simulink model "pendulum"  (R2022b)
settings: Solver=VariableStepAuto  StartTime=0.0  StopTime=100  RelTol=1e-3
StartFcn:
  | OpenAnimation;
undefined symbols (not defined in the file or in its folder): figId
libraries: aerolibanimutils x1
settings Model: Creator=l.ribeiro-lustosa  LastModifiedBy=fades
settings DebuggingCC: UnconnectedInputMsg=warning  UnconnectedOutputMsg=warning  UnconnectedLineMsg=warning
settings ModelReferenceCC: EnableRefExpFcnMdlSchedulingChecks=on
settings RTWCC: DLArmComputeVersion=19.05

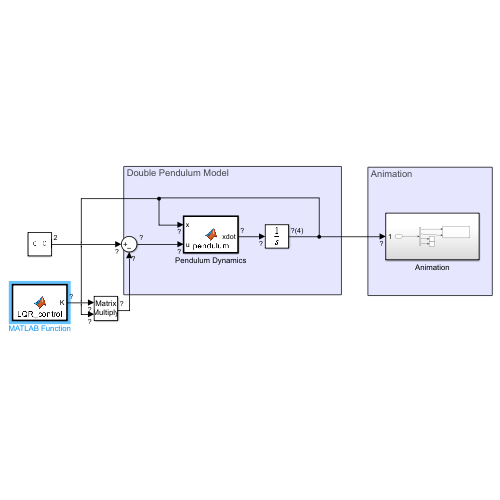
[thumbnail: Simulink's stored preview of the top-level diagram]
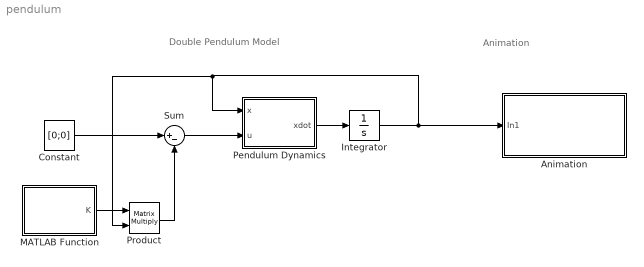
== system pendulum ==
  note: Animation
  note: Double Pendulum Model
  Animation : Subsystem
  Constant : Constant  Value=[0;0]
  Integrator : Integrator  InitialCondition=[175*pi/180;-5*pi/180;0;0]
  MATLAB Function : MATLAB Function  TreatAsAtomicUnit=on
  Pendulum Dynamics : MATLAB Function  TreatAsAtomicUnit=on
  Product : Product  Multiplication=Matrix(*)
  Sum : Sum  Inputs=|+-
  wires:
  Pendulum Dynamics/1(xdot) -> Integrator/1
  Integrator/1 -> Animation/1(In1), Product/2, Pendulum Dynamics/1(x)
  MATLAB Function/1(K) -> Product/1
  Product/1 -> Sum/2
  Sum/1 -> Pendulum Dynamics/2(u)
  Constant/1 -> Sum/1

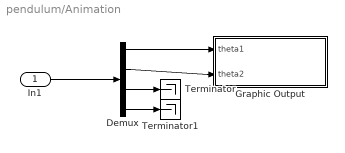
== system pendulum/Animation ==
  In1 : Inport
  Demux : Demux
  Graphic Output : Subsystem
  Terminator : Terminator
  Terminator1 : Terminator
  wires:
  Demux/4 -> Terminator1/1
  Demux/3 -> Terminator/1
  In1/1 -> Demux/1
  Demux/2 -> Graphic Output/2(theta2)
  Demux/1 -> Graphic Output/1(theta1)

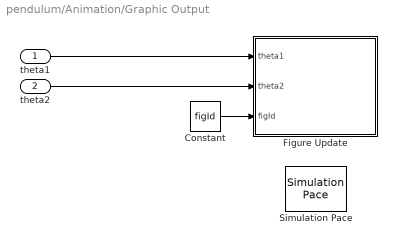
== system pendulum/Animation/Graphic Output ==
  theta1 : Inport
  theta2 : Inport  Port=2
  Constant : Constant  Value=figId
  Figure Update : MATLAB Function  TreatAsAtomicUnit=on
  Simulation Pace : aerolibanimutils/Simulation Pace  SimulationPace=1  SleepMode=Auto  OutputPaceError=off  SampleTime=1/30
  wires:
  Constant/1 -> Figure Update/3(figId)
  theta1/1 -> Figure Update/1(theta1)
  theta2/1 -> Figure Update/2(theta2)

== matlab function pendulum/Pendulum Dynamics ==
  data: x input; xdot output; u input
function xdot = pendulum(x,u)

xdot = double_pendulum(x,u);

== matlab function pendulum/MATLAB Function ==
  data: K output
function K = LQR_control()

n=4;
A = zeros(n,n);
B = zeros(n,2);
epsilon = 1e-6;

x_trim = [pi ; 0 ; 0 ; 0];
u_trim = [0 ; 0];

% A matrix
for k = 1:n
dx = zeros(n,1);
dx(k) = epsilon;
A(:,k) = imag(double_pendulum(x_trim+dx,u_trim))/epsilon;
end

% B matrix
for k = 1:2
du = [0 ; 0];
du(k) = epsilon;
B(:,k) = imag(double_pendulum(x_trim,u_trim+du))/epsilon;
end

Q = eye(4);
R = eye(2);
K = lqr(A,B,Q,R);

== matlab function pendulum/Animation/Graphic Output/Figure Update ==
  data: theta1 input; theta2 input; figId input
function updateFigure(theta1, theta2, figId)

L = 1;

% drawing rod
dx1 = [0;L*sin(theta1)];
dy1 = [0;-L*cos(theta1)];
UpdatePlot(figId,'rod1',dx1,dy1);
dx2 = [L*sin(theta1);L*sin(theta1)+L*sin(theta1+theta2)];
dy2 = [-L*cos(theta1);-L*cos(theta1)-L*cos(theta1+theta2)];
UpdatePlot(figId,'rod2',dx2,dy2);
% drawing pendulum ball
dx = [L*sin(theta1)];
dy = [-L*cos(theta1)];
UpdatePlot(figId,'ball1',dx,dy);
dx = [L*sin(theta1)+L*sin(theta1+theta2)];
dy = [-L*cos(theta1)-L*cos(theta1+theta2)];
UpdatePlot(figId,'ball2',dx,dy);

drawnow;

end

function UpdatePlot(hFig, plotTag, xData, yData)
    plotTarget = findobj(hFig, 'Tag', plotTag);
    set(plotTarget, 'XData', xData);
    set(plotTarget, 'YData', yData);
end
